simulink model "Lab7_Ex1_Template_gr2159"  (R2020a)
settings: Solver=ode1  StartTime=0.0  StopTime=90  FixedStep=0.002  RelTol=1e-3  EnableMultiTasking=on
libraries: quarc_library x3
settings Model: ExtModeTrigDuration=10000  Creator=merii  LastModifiedBy=Admin
settings SolverCC: PositivePriorityOrder=on
settings DataIOCC: ReturnWorkspaceOutputs=off
settings OptimizationCC: LifeSpan=inf
settings DebuggingCC: ArithmeticOperatorsInVariantConditions=warning
settings SFSimCC: SimUseLocalCustomCode=off  CustomCodeUndefinedFunction=UseInterfaceOnly
settings RTWCC: Description=QUARC Win64 Target  SystemTargetFile=quarc_win64.tlc  TemplateMakefile=quarc_default_tmf  RTWUseLocalCustomCode=off
settings CodeAppCC: StateflowObjectComments=on
settings STFCustomTargetCC: TargetPreCompLibLocation=C:\PROGRA~3\QUARC\lib\2020a\win64\release  TargetLangStandard=C99 (ISO)  ConcurrentExecutionCompliant=on  GRTInterface=on  SystemTargetFile=quarc_win64.tlc
settings GRTTargetCC: TargetPreCompLibLocation=C:\PROGRA~3\QUARC\lib\2020a\win64\release  ParMdlRefBuildCompliant=off  CompOptLevelCompliant=off  CombineOutputUpdateFcns=off  MatFileLogging=off  CPPClassGenCompliant=off  GRTInterface=on  UseToolchainInfoCompliant=off  ExtMode=on  ExtModeMexFile=quarc_comm
settings ConfigComp: CovMetricSettings=dswe

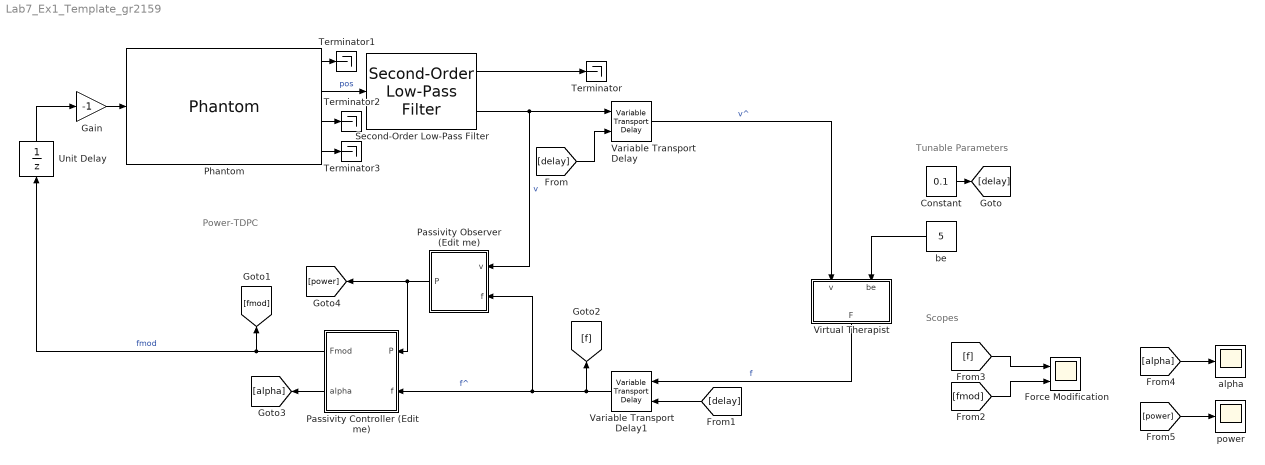
== system Lab7_Ex1_Template_gr2159 ==
  note: Power-TDPC
  note: Scopes
  note: Tunable Parameters
  Constant : Constant  Value=0.1
  Force Modification : Scope  NumInputPorts=2
  Gain : Gain  Gain=-1
  Passivity Controller (Edit me) : MATLAB Function  TreatAsAtomicUnit=on
  Passivity Observer (Edit me) : MATLAB Function  TreatAsAtomicUnit=on
  Phantom : quarc_library/Devices/Third-Party/SensAble/Phantom/Phantom  device_name=Default Device  output_type=Positions and Gimbal Angles  input_type=Cartesian space  velocity_limit_option=on  velocity_limit=1200  is_7dof=off  sample_time=-1
      settings: AttributesFormatString=(%<device_name>)  SourceProductName=QUARC Targets
  Second-Order Low-Pass Filter : quarc_library/Continuous/Second-Order Low-Pass Filter  params_source=Internal (dialog parameters)  input_width=50  input_zeta=1  input_init=0
  Terminator{,1..3} (4 alike) : Terminator
  Unit Delay : UnitDelay  SampleTime=-1  HasFrameUpgradeWarning=on
  Variable Transport Delay : VariableTransportDelay  MaximumDelay=10  ZeroDelay=on
  Variable Transport Delay1 : VariableTransportDelay  MaximumDelay=10  ZeroDelay=on
  Virtual Therapist : Subsystem
  alpha : Scope
  be : Constant  Value=5
  power : Scope
  wires:
  Phantom/2 -> Second-Order Low-Pass Filter/1  "pos"
  Second-Order Low-Pass Filter/2 -> Passivity Observer (Edit me)/1(v), Variable Transport Delay/1  "v"
  be/1 -> Virtual Therapist/2("be ")
  Second-Order Low-Pass Filter/1 -> Terminator/1
  Variable Transport Delay/1 -> Virtual Therapist/1(v)  "v^"
  Virtual Therapist/1(F) -> Variable Transport Delay1/1  "f"
  Constant/1 -> [delay]
  [delay] -> Variable Transport Delay/2
  [delay] -> Variable Transport Delay1/2
  Variable Transport Delay1/1 -> Passivity Controller (Edit me)/2(f), Passivity Observer (Edit me)/2(f), [f]  "f^"
  Gain/1 -> Phantom/1
  Unit Delay/1 -> Gain/1
  Passivity Controller (Edit me)/1(Fmod) -> [fmod], Unit Delay/1  "fmod"
  Passivity Controller (Edit me)/2(alpha) -> [alpha]
  Passivity Observer (Edit me)/1(P) -> [power], Passivity Controller (Edit me)/1(P)
  [fmod] -> Force Modification/2
  [f] -> Force Modification/1
  Phantom/1 -> Terminator1/1
  Phantom/3 -> Terminator2/1
  Phantom/4 -> Terminator3/1
  [alpha] -> alpha/1
  [power] -> power/1

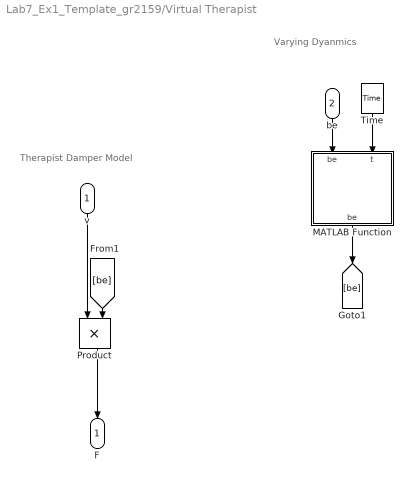
== system Lab7_Ex1_Template_gr2159/Virtual Therapist ==
  note: Therapist Damper Model
  note: Varying Dyanmics
  v : Inport
  "be " : Inport  Port=2
  MATLAB Function : MATLAB Function  TreatAsAtomicUnit=on
  Product : Product
  Time : quarc_library/Sources/Time/Time  time_source=Wall clock  sample_time=qc_get_step_size
  F : Outport
  wires:
  Time/1 -> MATLAB Function/2(t)
  MATLAB Function/1(be) -> [be]
  "be "/1 -> MATLAB Function/1("be ")
  Product/1 -> F/1
  v/1 -> Product/1
  [be] -> Product/2

== matlab function Lab7_Ex1_Template_gr2159/Passivity Controller (Edit me) ==
  data: Fmod output; P input; f input; alpha output
function [Fmod, alpha] = PC(P,f)
alpha = 0;
if P >= 0
    alpha = 1;
end
Fmod = alpha*f;
end

== matlab function Lab7_Ex1_Template_gr2159/Virtual Therapist/MATLAB Function ==
  data: be input; t input; be output
function be = fcn(be, t)

if t <= 30 %no therapy
    be = 0;
elseif t>=60 %resistive therapy
    be = -be; %assistive therapy
end

== matlab function Lab7_Ex1_Template_gr2159/Passivity Observer (Edit me) ==
  data: v input; f input; P output
function P = PO(v,f)

P = f' * v;

end
